simulink model "dataget_continuous"  (R2022a)
settings: Solver=VariableStepAuto  StartTime=0.0  StopTime=10.0  RelTol=1e-3
values from neighbouring files (symbols this model uses):
  sam_time = 40    [code_tra.m]
  seed = 17    [code_tra.m]
  ts = 0.05    [code_tra.m]
undefined symbols (not defined in the file or in its folder): A0, B0, C0, D0
settings Model: Creator=IDS_PC  LastModifiedBy=IDS_PC

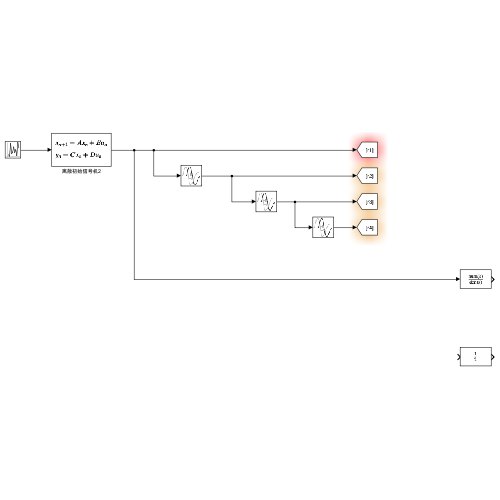
[thumbnail: Simulink's stored preview of the top-level diagram]
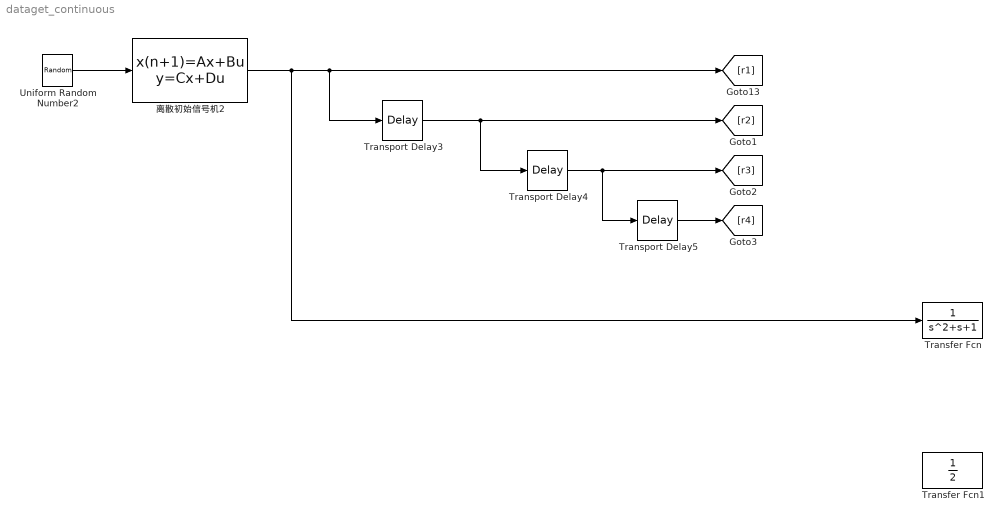
== system dataget_continuous ==
  Transfer Fcn : TransferFcn  Denominator=[1 1 1]
  Transfer Fcn1 : TransferFcn  Denominator=[2]
  Transport Delay3 : TransportDelay  DelayTime=ts
  Transport Delay4 : TransportDelay  DelayTime=ts
  Transport Delay5 : TransportDelay  DelayTime=ts
  Uniform Random Number2 : UniformRandomNumber  Minimum=0  Maximum=10  Seed=seed  SampleTime=sam_time
  离散初始信号机2 : DiscreteStateSpace  A=A0  B=B0  C=C0  D=D0  SampleTime=ts
  wires:
  Uniform Random Number2/1 -> 离散初始信号机2/1
  离散初始信号机2/1 -> Transfer Fcn/1, Transport Delay3/1, [r1]
  Transport Delay3/1 -> [r2], Transport Delay4/1
  Transport Delay4/1 -> Transport Delay5/1, [r3]
  Transport Delay5/1 -> [r4]
